simulink model "task1_5"  (R2020b)
settings: Solver=VariableStepAuto  StartTime=0.0  StopTime=10.0  RelTol=1e-3
libraries: simulink x1
settings Model: Creator=zceexdu  LastModifiedBy=zceexdu

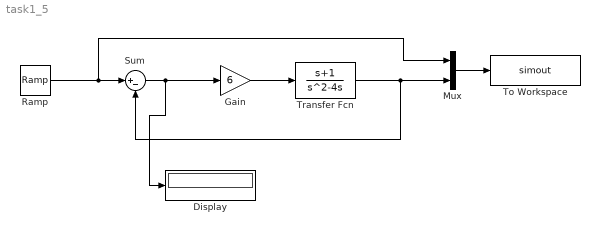
== system task1_5 ==
  Display : Display
  Gain : Gain  Gain=6
  Mux : Mux  Inputs=2
  Ramp : simulink/Sources/Ramp  slope=1  start=0  InitialOutput=0
  Sum : Sum  Inputs=|+-
  To Workspace : ToWorkspace  VariableName=simout  SaveFormat=Timeseries  SampleTime=-1
  Transfer Fcn : TransferFcn  Numerator=[1 1]  Denominator=[1 -4 0]
  wires:
  Sum/1 -> Display/1, Gain/1
  Gain/1 -> Transfer Fcn/1
  Transfer Fcn/1 -> Sum/2, Mux/2
  Ramp/1 -> Mux/1, Sum/1
  Mux/1 -> To Workspace/1
